simulink model "UAV_CL"  (R2021b)
settings: Solver=FixedStepAuto  StartTime=0.0  StopTime=20  FixedStep=0.001  RelTol=1e-3
InitFcn:
  | param
values from neighbouring files (symbols this model uses):
  P = [-0.6408, 0.37, 0.6408, -0.37; -0.37, -0.6408, 0.37, 0.6408; 0.002*((s+0.1)^2), 0.002*((s+0.1)^2), 0.002*((s+0.1)^2), 0.002*((s+0.1)^2); -0.25*((s+0.1)^2), 0.25*((s+0.1)^2), -0.25*((s+0.1)^2), 0.25*((s+0.1)^2)]    [quadrotor_plant.m]    (also in youla_controller.m; youlascripts.m = [-0.6408, 0.37, 0.6408, -0.37; -0.37, -0.6408, 0.37, 0.6408;)
undefined symbols (not defined in the file or in its folder): autopilot, drawAircraft, forces_moments, plotmavstatevariables
settings Model: Creator=beard  LastModifiedBy=yuankaizhu
settings SolverCC: AlgebraicLoopSolver=TrustRegion
settings DataIOCC: LimitDataPoints=on  SaveFormat=Array  ReturnWorkspaceOutputs=off
settings OptimizationCC: BlockReduction=off  BooleanDataType=off  LifeSpan=inf
settings DebuggingCC: SaveWithParameterizedLinksMsg=none  UnderspecifiedInitializationDetection=Classic  MergeDetectMultiDrivingBlocksExec=none  SignalResolutionControl=TryResolveAllWithWarning  SFUnexpectedBacktrackingDiag=warning  SFNoUnconditionalDefaultTransitionDiag=warning  SFExecutionAtInitializationDiag=none  SFMachineParentedDataDiag=warning  ArithmeticOperatorsInVariantConditions=warning
settings HardwareCC: ProdBitPerPointer=32  ProdBitPerSizeT=32  ProdBitPerPtrDiffT=32  ProdLargestAtomicFloat=None  ProdIntDivRoundTo=Undefined  ProdEndianess=Unspecified  ProdWordSize=32  ProdHWDeviceType=32-bit Generic  TargetUnknown=on
settings ModelReferenceCC: PropagateSignalLabelsOutOfModel=off
settings SFSimCC: SimUseLocalCustomCode=off  CustomCodeUndefinedFunction=UseInterfaceOnly
settings RTWCC: RTWUseLocalCustomCode=off
settings CodeAppCC: StateflowObjectComments=on
settings GRTTargetCC: TargetLangStandard=C89/C90 (ANSI)
settings ConfigComp: CovMetricSettings=dw  CovSaveCumulativeToWorkspaceVar=on  CovSaveSingleToWorkspaceVar=on  CovExternalEMLEnable=off  CovSFcnEnable=off

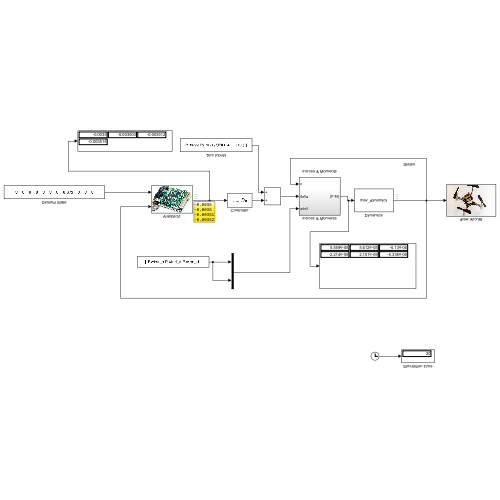
[thumbnail: Simulink's stored preview of the top-level diagram]
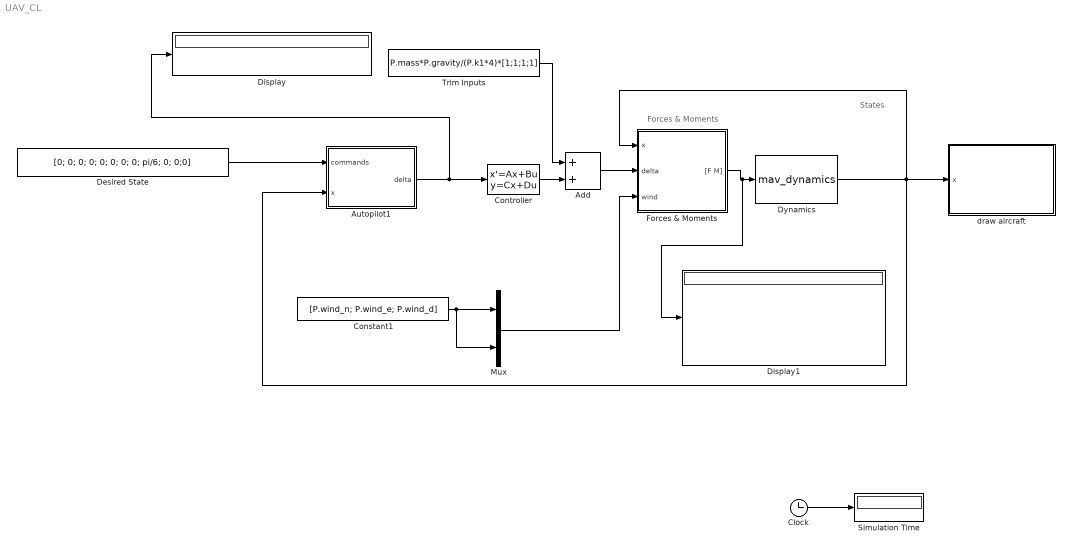
== system UAV_CL ==
  note: States
  note: Forces & Moments
  Add : Sum
  Autopilot1 : Subsystem
      mask Display: image(imread('kestrel.jpg'))
  Clock : Clock
  Constant1 : Constant  Value=[P.wind_n; P.wind_e; P.wind_d]
  Controller : StateSpace  A=P.K.A  B=P.K.B  C=P.K.C  D=P.K.D  InitialCondition=0
  Desired State : Constant  Value=[0; 0; 0; 0; 0; 0; 0; 0; pi/6; 0; 0;0]
  Display : Display
  Display1 : Display
  Dynamics : S-Function  FunctionName=mav_dynamics  Parameters=P,0  SFunctionDeploymentMode=off  EnableBusSupport=off
  Forces & Moments : Subsystem
  Mux : Mux  Inputs=2
  Simulation Time : Display
  Trim Inputs : Constant  Value=P.mass*P.gravity/(P.k1*4)*[1;1;1;1]
  draw aircraft : Subsystem
      mask Display: image(imread('crazyflie.jpg'))
  wires:
  Dynamics/1 -> Autopilot1/2(x), Forces & Moments/1(x), draw aircraft/1(x)
  Desired State/1 -> Autopilot1/1(commands)
  Forces & Moments/1("[F M]") -> Display1/1, Dynamics/1
  Constant1/1 -> Mux/2, Mux/1
  Mux/1 -> Forces & Moments/3(wind)
  Clock/1 -> Simulation Time/1
  Autopilot1/1(delta) -> Controller/1, Display/1
  Add/1 -> Forces & Moments/2(delta)
  Trim Inputs/1 -> Add/1
  Controller/1 -> Add/2

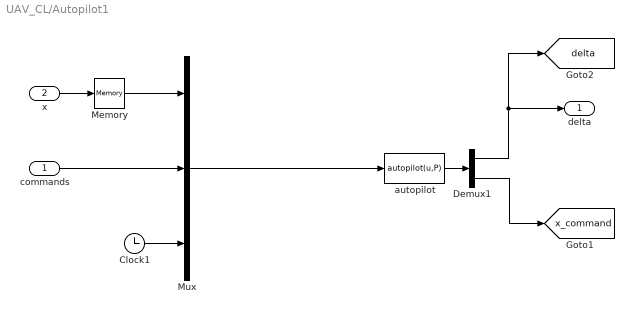
== system UAV_CL/Autopilot1 ==
  commands : Inport
  x : Inport  Port=2
  Clock1 : Clock
  Demux1 : Demux  Outputs=[4 12]
  Memory : Memory
  Mux : Mux  Inputs=3
  autopilot : MATLABFcn  MATLABFcn=autopilot(u,P)  OutputDimensions=16  SampleTime=P.Ts
  delta : Outport
  tag scope: delta=global, x_command=global
  wires:
  commands/1 -> Mux/2
  Clock1/1 -> Mux/3
  autopilot/1 -> Demux1/1
  Demux1/1 -> [delta], delta/1
  Demux1/2 -> [x_command]
  x/1 -> Memory/1
  Memory/1 -> Mux/1
  Mux/1 -> autopilot/1

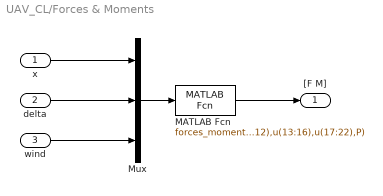
== system UAV_CL/Forces & Moments ==
  x : Inport
  delta : Inport  Port=2
  wind : Inport  Port=3
  MATLAB Fcn : MATLABFcn  MATLABFcn=forces_moments(u(1:12),u(13:16),u(17:22),P)  OutputDimensions=6
  Mux : Mux  Inputs=3
  "[F M]" : Outport
  wires:
  x/1 -> Mux/1
  delta/1 -> Mux/2
  wind/1 -> Mux/3
  MATLAB Fcn/1 -> "[F M]"/1
  Mux/1 -> MATLAB Fcn/1

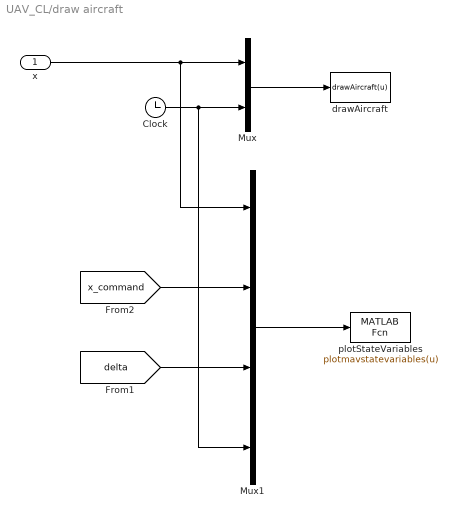
== system UAV_CL/draw aircraft ==
  x : Inport
  Clock : Clock
  Mux : Mux  Inputs=2
  Mux1 : Mux
  drawAircraft : MATLABFcn  MATLABFcn=drawAircraft(u)  OutputDimensions=0  SampleTime=0.1
  plotStateVariables : MATLABFcn  MATLABFcn=plotmavstatevariables(u)  OutputDimensions=0  SampleTime=0.1
  wires:
  Mux1/1 -> plotStateVariables/1
  Clock/1 -> Mux1/4, Mux/2
  x/1 -> Mux1/1, Mux/1
  Mux/1 -> drawAircraft/1
  [x_command] -> Mux1/2
  [delta] -> Mux1/3
